simulink model "fixedEEControlR2016a"  (Simulink 8.7)
settings: Solver=ode5  StartTime=0.0  StopTime=30  FixedStep=0.01  RelTol=1e-3
values from neighbouring files (symbols this model uses):
  CONFIG =     [matlab_working.mat]
libraries: WBToolboxLibrary x13
settings Model: Creator=yeshi  LastModifiedBy=yeshi
settings DataIOCC: LimitDataPoints=off  SaveFormat=Dataset
settings DebuggingCC: UnderspecifiedInitializationDetection=Simplified  MergeDetectMultiDrivingBlocksExec=error
settings HardwareCC: ProdBitPerPointer=64  ProdLargestAtomicFloat=Float  ProdIntDivRoundTo=Zero  ProdEndianess=LittleEndian  ProdWordSize=64  ProdHWDeviceType=Intel->x86-64 (Windows64)
settings ModelReferenceCC: PropagateSignalLabelsOutOfModel=on
settings ConfigComp: CovModelRefEnable=off

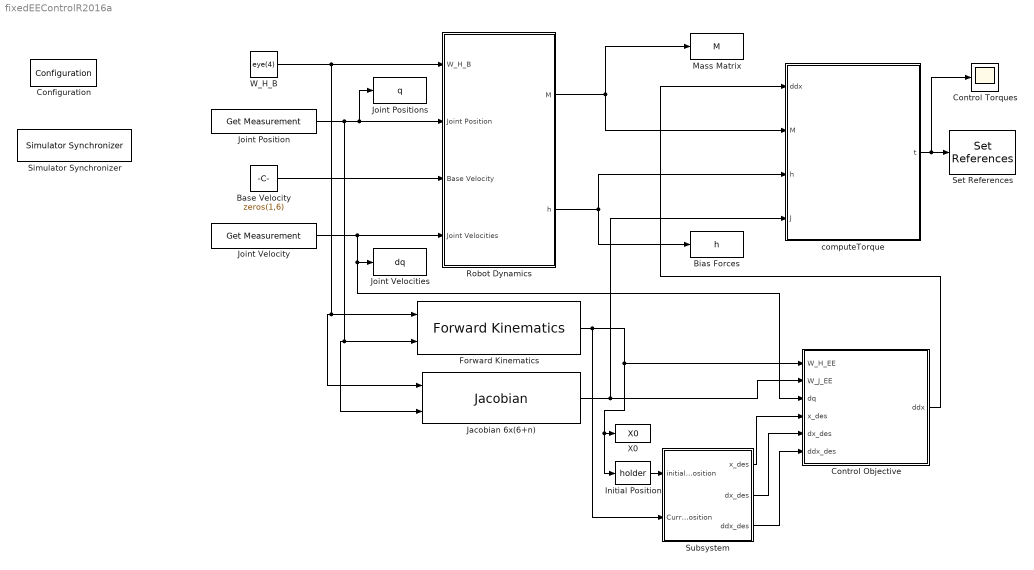
== system fixedEEControlR2016a ==
  "Base Velocity " : Constant  Value=zeros(1,6)
  Bias Forces : ToWorkspace  VariableName=h  SaveFormat=Timeseries  SampleTime=-1
  Configuration : WBToolboxLibrary/Utilities/Configuration  ConfigSource=Workspace  ConfigObject='WBTConfigRobot'
  Control Torques : Scope
  Control Objective : MATLAB Function  TreatAsAtomicUnit=on
  Forward Kinematics : WBToolboxLibrary/wholeBodyModel/Kinematics/Forward Kinematics  frameName=CONFIG.EE
  "Initial Position " : WBToolboxLibrary/Utilities/holder 
  Jacobian 6x(6+n) : WBToolboxLibrary/wholeBodyModel/Jacobians/Jacobian  frameName=CONFIG.EE
  Joint Position : WBToolboxLibrary/wholeBodyStates/Get Measurement  measuredType=Joints Position
  "Joint Positions " : ToWorkspace  VariableName=q  SaveFormat=Timeseries  SampleTime=-1
  Joint Velocities : ToWorkspace  VariableName=dq  SaveFormat=Timeseries  SampleTime=-1
  Joint Velocity : WBToolboxLibrary/wholeBodyStates/Get Measurement  measuredType=Joints Velocity
  "Mass Matrix " : ToWorkspace  VariableName=M  SaveFormat=Timeseries  SampleTime=-1
  Robot Dynamics : Subsystem
  Set References : WBToolboxLibrary/wholeBodyActuators/Set References  controlType=Torque  refSpeed=50
  Simulator Synchronizer : WBToolboxLibrary/Utilities/Simulator Synchronizer  period=0.01  serverPortName='/clock/rpc'  clientPortName='/WBT_synchronizer/rpc:o'
  Subsystem : Subsystem
  "W_H_B " : Constant  Value=eye(4)
  X0 : ToWorkspace  VariableName=X0  SaveFormat=Timeseries  SampleTime=-1
  computeTorque : MATLAB Function  TreatAsAtomicUnit=on
  wires:
  Joint Position/1 -> "Joint Positions "/1, Robot Dynamics/2(Joint Position), Jacobian 6x(6+n)/2, Forward Kinematics/2
  Joint Velocity/1 -> Control Objective/3(dq), Joint Velocities/1, Robot Dynamics/4(" Joint Velocities ")
  "W_H_B "/1 -> Jacobian 6x(6+n)/1, Forward Kinematics/1, Robot Dynamics/1(W_H_B)
  "Base Velocity "/1 -> Robot Dynamics/3(Base Velocity)
  Robot Dynamics/1(M) -> computeTorque/2(M), "Mass Matrix "/1
  computeTorque/1(t) -> Control Torques/1, Set References/1
  Robot Dynamics/2(h) -> computeTorque/3(h), Bias Forces/1
  Jacobian 6x(6+n)/1 -> computeTorque/4(J), Control Objective/2(W_J_EE)
  Control Objective/1(ddx) -> computeTorque/1(ddx)
  Subsystem/1(x_des) -> Control Objective/4(x_des)
  Subsystem/2(dx_des) -> Control Objective/5(dx_des)
  Subsystem/3(ddx_des) -> Control Objective/6(ddx_des)
  Forward Kinematics/1 -> Subsystem/2(Current Position), Control Objective/1(W_H_EE), "Initial Position "/1, X0/1
  "Initial Position "/1 -> Subsystem/1(initial Position)

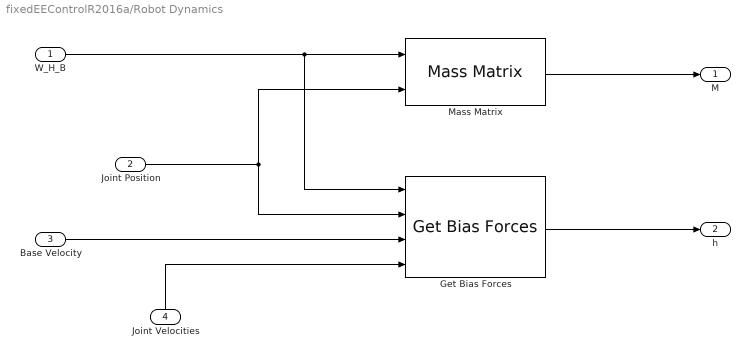
== system fixedEEControlR2016a/Robot Dynamics ==
  W_H_B : Inport
  Joint Position : Inport  Port=2
  Base Velocity : Inport  Port=3
  " Joint Velocities " : Inport  Port=4
  Get Bias Forces : WBToolboxLibrary/wholeBodyModel/Dynamics/Get Bias Forces
  Mass Matrix : WBToolboxLibrary/wholeBodyModel/Dynamics/Mass Matrix
  M : Outport
  h : Outport  Port=2
  wires:
  Joint Position/1 -> Mass Matrix/2, Get Bias Forces/2
  " Joint Velocities "/1 -> Get Bias Forces/4
  Mass Matrix/1 -> M/1
  Get Bias Forces/1 -> h/1
  W_H_B/1 -> Get Bias Forces/1, Mass Matrix/1
  Base Velocity/1 -> Get Bias Forces/3

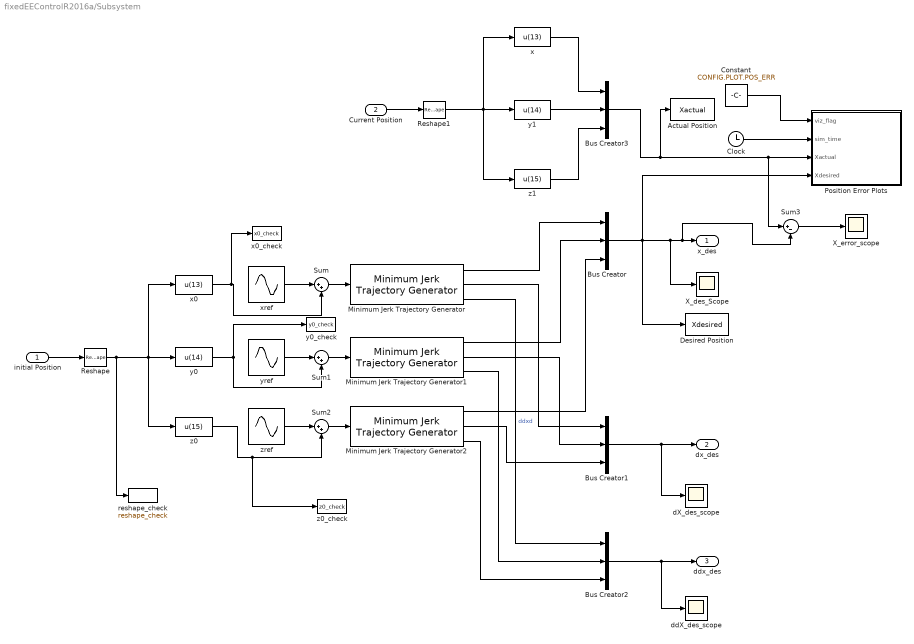
== system fixedEEControlR2016a/Subsystem ==
  initial Position : Inport
  Current Position : Inport  Port=2
  Actual Position : ToWorkspace  VariableName=Xactual  SaveFormat=Timeseries  SampleTime=-1
  Bus Creator{,1..3} (4 alike) : BusCreator  Inputs=3
  Clock : Clock
  Constant : Constant  Value=CONFIG.PLOT.POS_ERR
  Desired Position : ToWorkspace  VariableName=Xdesired  SaveFormat=Timeseries  SampleTime=-1
  Minimum Jerk Trajectory Generator : WBToolboxLibrary/Utilities/Minimum Jerk Trajectory Generator  externalSettlingTime=off  settlingTime=3  sampleTime=0.01  resetOnSettlingTime=off  firstDerivatives=on  secondDerivatives=on  explicitInitialValue=off
  Minimum Jerk Trajectory Generator1 : WBToolboxLibrary/Utilities/Minimum Jerk Trajectory Generator  externalSettlingTime=off  settlingTime=3  sampleTime=0.01  resetOnSettlingTime=off  firstDerivatives=on  secondDerivatives=on  explicitInitialValue=off
  Minimum Jerk Trajectory Generator2 : WBToolboxLibrary/Utilities/Minimum Jerk Trajectory Generator  externalSettlingTime=off  settlingTime=3  sampleTime=0.01  resetOnSettlingTime=off  firstDerivatives=on  secondDerivatives=on  explicitInitialValue=off
  "Position Error Plots " : MATLAB Function  TreatAsAtomicUnit=on
  Reshape : Reshape
  Reshape1 : Reshape
  Sum : Sum  Inputs=|++
  Sum1 : Sum  Inputs=|++
  Sum2 : Sum  Inputs=|++
  Sum3 : Sum  Inputs=|+-
  X_des_Scope : Scope
  X_error_scope : Scope
  dX_des_scope : Scope
  ddX_des_scope : Scope
  reshape_check : ToWorkspace  VariableName=reshape_check  SaveFormat=Timeseries  SampleTime=-1
  x : Fcn  Expr=u(13)
  x0 : Fcn  Expr=u(13)
  x0_check : ToWorkspace  VariableName=x0_check  SaveFormat=Timeseries  SampleTime=-1
  xref : Sin  Amplitude=0  SampleTime=0
  y0 : Fcn  Expr=u(14)
  y0_check : ToWorkspace  VariableName=y0_check  SaveFormat=Timeseries  SampleTime=-1
  y1 : Fcn  Expr=u(14)
  yref : Sin  Amplitude=0.2  SampleTime=0
  z0 : Fcn  Expr=u(15)
  z0_check : ToWorkspace  VariableName=z0_check  SaveFormat=Timeseries  SampleTime=-1
  z1 : Fcn  Expr=u(15)
  zref : Sin  Amplitude=0.2  Phase=pi/2  SampleTime=0
  x_des : Outport
  dx_des : Outport  Port=2
  ddx_des : Outport  Port=3
  wires:
  Minimum Jerk Trajectory Generator2/2 -> Bus Creator1/3
  Sum2/1 -> Minimum Jerk Trajectory Generator2/1
  Minimum Jerk Trajectory Generator2/1 -> Bus Creator/3
  Minimum Jerk Trajectory Generator/3 -> Bus Creator2/1  "ddxd"
  yref/1 -> Sum1/1
  Minimum Jerk Trajectory Generator/1 -> Bus Creator/1
  Minimum Jerk Trajectory Generator1/3 -> Bus Creator2/2
  y0/1 -> Sum1/2, y0_check/1
  Sum1/1 -> Minimum Jerk Trajectory Generator1/1
  Minimum Jerk Trajectory Generator2/3 -> Bus Creator2/3
  Bus Creator1/1 -> dx_des/1, dX_des_scope/1
  zref/1 -> Sum2/1
  Minimum Jerk Trajectory Generator1/2 -> Bus Creator1/2
  Bus Creator2/1 -> ddx_des/1, ddX_des_scope/1
  Bus Creator/1 -> Desired Position/1, "Position Error Plots "/4(Xdesired), Sum3/2, x_des/1, X_des_Scope/1
  Minimum Jerk Trajectory Generator1/1 -> Bus Creator/2
  xref/1 -> Sum/1
  Minimum Jerk Trajectory Generator/2 -> Bus Creator1/1
  Sum/1 -> Minimum Jerk Trajectory Generator/1
  z0/1 -> z0_check/1, Sum2/2
  Reshape/1 -> reshape_check/1, z0/1, x0/1, y0/1
  x0/1 -> x0_check/1, Sum/2
  initial Position/1 -> Reshape/1
  Current Position/1 -> Reshape1/1
  Reshape1/1 -> z1/1, x/1, y1/1
  x/1 -> Bus Creator3/1
  y1/1 -> Bus Creator3/2
  z1/1 -> Bus Creator3/3
  Clock/1 -> "Position Error Plots "/2(sim_time)
  Bus Creator3/1 -> Actual Position/1, Sum3/1, "Position Error Plots "/3(Xactual)
  Constant/1 -> "Position Error Plots "/1(viz_flag)
  Sum3/1 -> X_error_scope/1

== matlab function Control Objective ==
  data: W_H_EE input double; ddx output double; W_J_EE input double; dq input double; x_des input double; dx_des input double; ddx_des input double
function ddx = controlObjective(W_H_EE,W_J_EE,dq,x_des,dx_des,ddx_des)
   
    x = W_H_EE(1:3,4)-x_des;
    dx = W_J_EE(1:3,7:end)*dq-dx_des;
   
    Kp = [100;100;100];
    Kd = [1;1;1];

    ddx = ddx_des-Kp.*x-Kd.*dx; 

end

== matlab function computeTorque ==
  data: ddx input double; M input double; h input double; t output double; J input double
function t = computeTorque(ddx,M,h,J)
%#codegen
% t = M*inv(J)*ddx+h

v1 = M*pinv(J);
v2 = v1(:,1:3)*ddx + h;
t = v2(7:end);

end

== matlab function Subsystem/Position Error Plots  ==
  data: viz_flag input double; sim_time input double; Xactual input double; Xdesired input double
function positionErrorPlots(viz_flag,sim_time,Xactual,Xdesired)
%#codegen

coder.extrinsic('animatedline')
coder.extrinsic('addpoints')
coder.extrinsic('legend')
coder.extrinsic('clearpoints')

if(viz_flag ~= 0)
    
    Xerror = Xactual - Xdesired;
    curve_position_error = animatedline('LineWidth',0.1,'Marker','+');

    if(sim_time == 0)
    
        clf;
        close;
    
        fig1 = figure;
        view(177,15); hold on;
        grid on;
        xlabel('x');
        ylabel('y');
        zlabel('z');
        title('Position Error'); hold on;
% %         axis([-0.3 0.3 -0.3 0.3 -0.3 0.3]);
       
    end
    
    figure(1);
    addpoints(curve_position_error,Xerror(1),Xerror(2),Xerror(3));
    drawnow;
    
end

end
